simulink model "torque_vectoring_model"  (R2019a)
settings: Solver=VariableStepAuto  StartTime=0.0  StopTime=20.0  RelTol=1e-3
undefined symbols (not defined in the file): h, l, w, wn
settings Model: Creator=jacoboffersen  LastModifiedBy=jacoboffersen

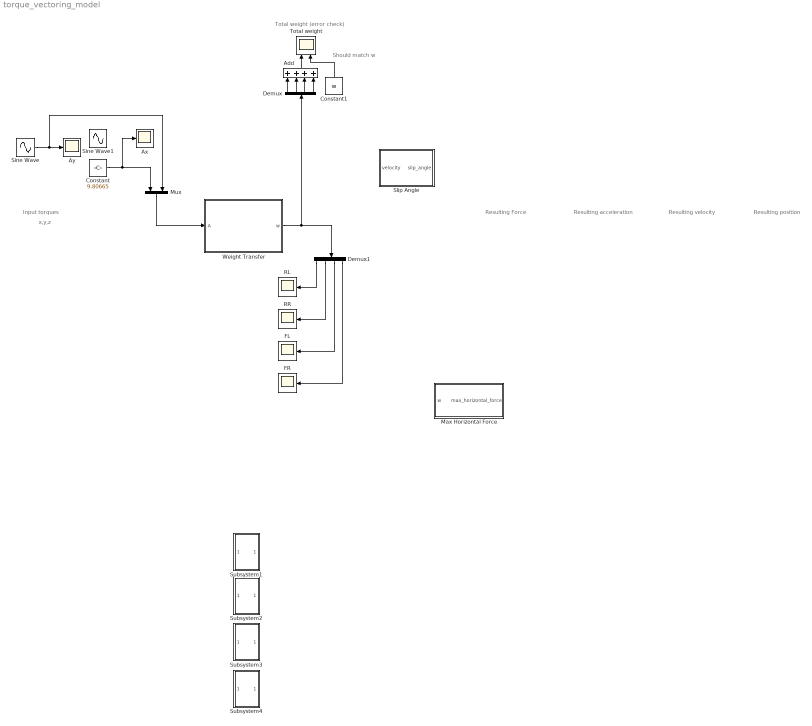
== system torque_vectoring_model ==
  note: x,y,z
  note: Resulting
      | acceleration
  note: Should match w
  note: Total weight (error check)
  note: Input torques
  note: Resulting
      | velocity
  note: Resulting
      | Force
  note: Resulting
      | position
  Add : Sum  Inputs=++++
  Ax : Scope
  Ay : Scope
  Constant : Constant  Value=9.80665
  Constant1 : Constant  Value=w
  Demux : Demux
  Demux1 : Demux
  FL : Scope
  FR : Scope
  Max Horizontal Force : Subsystem
  Mux : Mux  Inputs=2
  RL : Scope
  RR : Scope
  Sine Wave : Sin  Amplitude=9.80665  SampleTime=0
  Sine Wave1 : Sin  Amplitude=9.80665  SampleTime=0
  "Slip Angle " : Subsystem
  Subsystem1 : Subsystem
  Subsystem2 : Subsystem
  Subsystem3 : Subsystem
  Subsystem4 : Subsystem
  Total weight : Scope  NumInputPorts=2
  Weight Transfer : Subsystem
  wires:
  Sine Wave/1 -> Mux/2, Ay/1
  Constant/1 -> Mux/1, Ax/1
  Add/1 -> Total weight/1
  Demux/1 -> Add/1
  Demux/2 -> Add/2
  Demux/3 -> Add/3
  Demux/4 -> Add/4
  Mux/1 -> Weight Transfer/1(A)
  Constant1/1 -> Total weight/2
  Demux1/4 -> FR/1
  Demux1/3 -> FL/1
  Demux1/2 -> RR/1
  Demux1/1 -> RL/1
  Weight Transfer/1(w) -> Demux/1, Demux1/1

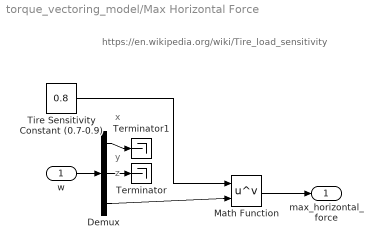
== system torque_vectoring_model/Max Horizontal Force ==
  note: https://en.wikipedia.org/wiki/Tire_load_sensitivity
  note: z
  note: y
  note: x
  w : Inport
  Demux : Demux  Outputs=3
  Math Function : Math  Operator=pow  SaturateOnIntegerOverflow=on
  Terminator : Terminator
  Terminator1 : Terminator
  Tire Sensitivity Constant (0.7-0.9) : Constant  Value=0.8
  max_horizontal_force : Outport
  wires:
  w/1 -> Demux/1
  Demux/3 -> Math Function/2
  Tire Sensitivity Constant (0.7-0.9)/1 -> Math Function/1
  Math Function/1 -> max_horizontal_force/1
  Demux/1 -> Terminator1/1
  Demux/2 -> Terminator/1

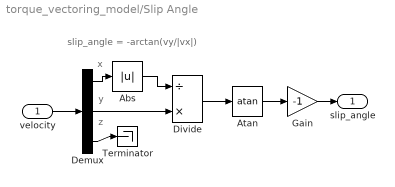
== system torque_vectoring_model/Slip Angle  ==
  note: slip_angle = -arctan(vy/|vx|)
  note: z
  note: y
  note: x
  velocity : Inport
  Abs : Abs
  Atan : Trigonometry  Operator=atan
  Demux : Demux  Outputs=3
  Divide : Product  Inputs=/*
  Gain : Gain  Gain=-1
  Terminator : Terminator
  slip_angle : Outport
  wires:
  velocity/1 -> Demux/1
  Gain/1 -> slip_angle/1
  Atan/1 -> Gain/1
  Divide/1 -> Atan/1
  Demux/1 -> Abs/1
  Abs/1 -> Divide/1
  Demux/2 -> Divide/2
  Demux/3 -> Terminator/1

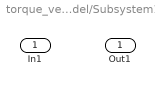
== system torque_vectoring_model/Subsystem1 ==
  In1 : Inport
  Out1 : Outport

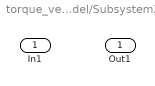
== system torque_vectoring_model/Subsystem2 ==
  In1 : Inport
  Out1 : Outport

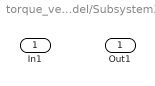
== system torque_vectoring_model/Subsystem3 ==
  In1 : Inport
  Out1 : Outport

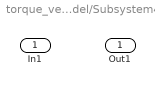
== system torque_vectoring_model/Subsystem4 ==
  In1 : Inport
  Out1 : Outport

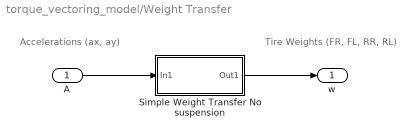
== system torque_vectoring_model/Weight Transfer ==
  note: Tire Weights (FR, FL, RR, RL)
  note: Accelerations (ax, ay)
  A : Inport
  Simple Weight Transfer No suspension : Subsystem
  w : Outport
  wires:
  A/1 -> Simple Weight Transfer No suspension/1(In1)
  Simple Weight Transfer No suspension/1(Out1) -> w/1

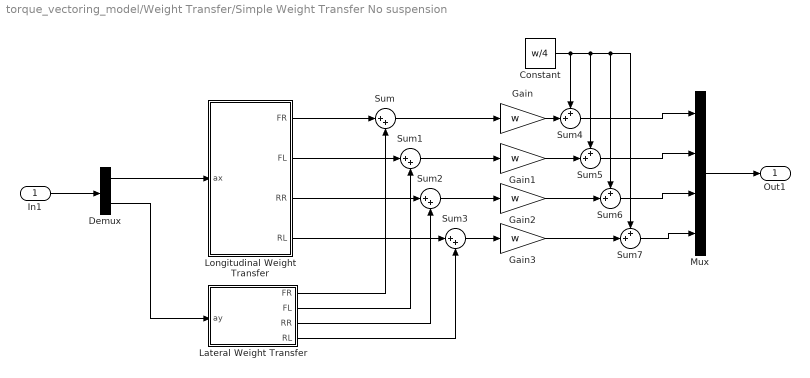
== system torque_vectoring_model/Weight Transfer/Simple Weight Transfer No suspension ==
  In1 : Inport
  Constant : Constant  Value=w/4
  Demux : Demux  Outputs=2
  Gain{,1..3} (4 alike) : Gain  Gain=w
  "Lateral Weight Transfer " : Subsystem
  Longitudinal Weight Transfer : Subsystem
  Mux : Mux
  Sum{,1..3} (4 alike) : Sum  Inputs=|++
  Sum{4..7} (4 alike) : Sum  Inputs=++|
  Out1 : Outport
  wires:
  Longitudinal Weight Transfer/4(RL) -> Sum3/1
  Sum/1 -> Gain/1
  "Lateral Weight Transfer "/4(RL) -> Sum3/2
  Sum1/1 -> Gain1/1
  "Lateral Weight Transfer "/1(FR) -> Sum/2
  Mux/1 -> Out1/1
  Longitudinal Weight Transfer/2(FL) -> Sum1/1
  In1/1 -> Demux/1
  Constant/1 -> Sum4/1, Sum5/1, Sum6/1, Sum7/1
  Longitudinal Weight Transfer/3(RR) -> Sum2/1
  Gain2/1 -> Sum6/2
  "Lateral Weight Transfer "/3(RR) -> Sum2/2
  Sum3/1 -> Gain3/1
  Gain/1 -> Sum4/2
  Sum2/1 -> Gain2/1
  Demux/1 -> Longitudinal Weight Transfer/1(ax)
  Gain1/1 -> Sum5/2
  Longitudinal Weight Transfer/1(FR) -> Sum/1
  Sum7/1 -> Mux/4
  Sum6/1 -> Mux/3
  Demux/2 -> "Lateral Weight Transfer "/1(ay)
  Sum5/1 -> Mux/2
  Gain3/1 -> Sum7/2
  "Lateral Weight Transfer "/2(FL) -> Sum1/2
  Sum4/1 -> Mux/1

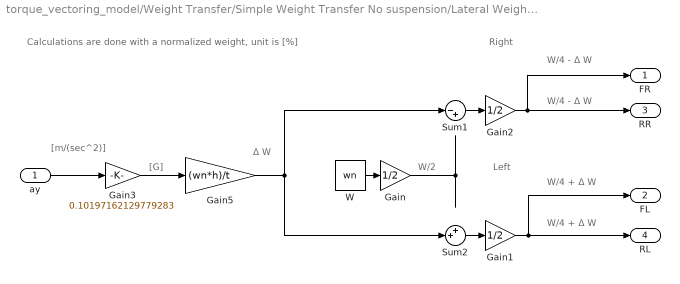
== system torque_vectoring_model/Weight Transfer/Simple Weight Transfer No suspension/Lateral Weight Transfer  ==
  note: Calculations are done with a normalized weight, unit is [%]
  note: [G]
  note: Left
  note: Right
  note: [m/(sec^2)]
  note: Δ W
  note: W/2
  note: W/4 - Δ W
  note: W/4 - Δ W
  note: W/4 + Δ W
  note: W/4 + Δ W
  ay : Inport
  Gain : Gain  Gain=1/2
  Gain1 : Gain  Gain=1/2
  Gain2 : Gain  Gain=1/2
  Gain3 : Gain  Gain=0.10197162129779283
  Gain5 : Gain  Gain=(wn*h)/t
  Sum1 : Sum  Inputs=|-+
  Sum2 : Sum  Inputs=++|
  W : Constant  Value=wn
  FR : Outport
  FL : Outport  Port=2
  RR : Outport  Port=3
  RL : Outport  Port=4
  wires:
  Sum1/1 -> Gain2/1
  Gain/1 -> ?
  Gain1/1 -> FL/1, RL/1
  Gain2/1 -> FR/1, RR/1
  Sum2/1 -> Gain1/1
  W/1 -> Gain/1
  Gain5/1 -> Sum1/1, Sum2/2
  ay/1 -> Gain3/1
  Gain3/1 -> Gain5/1

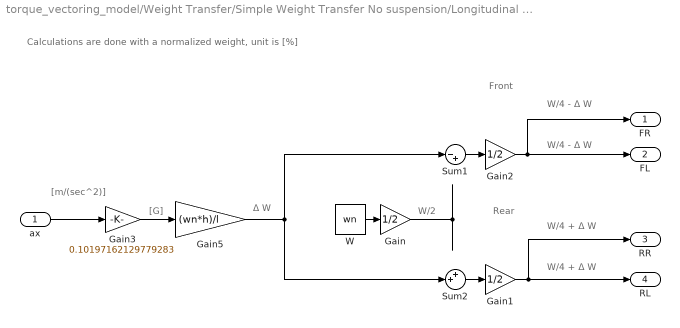
== system torque_vectoring_model/Weight Transfer/Simple Weight Transfer No suspension/Longitudinal Weight Transfer ==
  note: [G]
  note: Rear
  note: Front
  note: [m/(sec^2)]
  note: Δ W
  note: W/2
  note: W/4 - Δ W
  note: W/4 - Δ W
  note: W/4 + Δ W
  note: W/4 + Δ W
  note: Calculations are done with a normalized weight, unit is [%]
  ax : Inport
  Gain : Gain  Gain=1/2
  Gain1 : Gain  Gain=1/2
  Gain2 : Gain  Gain=1/2
  Gain3 : Gain  Gain=0.10197162129779283
  Gain5 : Gain  Gain=(wn*h)/l
  Sum1 : Sum  Inputs=|-+
  Sum2 : Sum  Inputs=++|
  W : Constant  Value=wn
  FR : Outport
  FL : Outport  Port=2
  RR : Outport  Port=3
  RL : Outport  Port=4
  wires:
  Sum1/1 -> Gain2/1
  Gain/1 -> ?
  Gain1/1 -> RR/1, RL/1
  Gain2/1 -> FL/1, FR/1
  Sum2/1 -> Gain1/1
  W/1 -> Gain/1
  Gain5/1 -> Sum1/1, Sum2/2
  ax/1 -> Gain3/1
  Gain3/1 -> Gain5/1
